simulink model "Control"  (R2022b)
settings: Solver=ode4  StartTime=0.0  StopTime=60  FixedStep=0.001  RelTol=1e-3
undefined symbols (not defined in the file): Am, gv, iPhi, NC, NCP, nodeControl, nodeDisturbe, Psi1, Psi2, V0, W1, W2
settings Model: Creator=raul  LastModifiedBy=raul

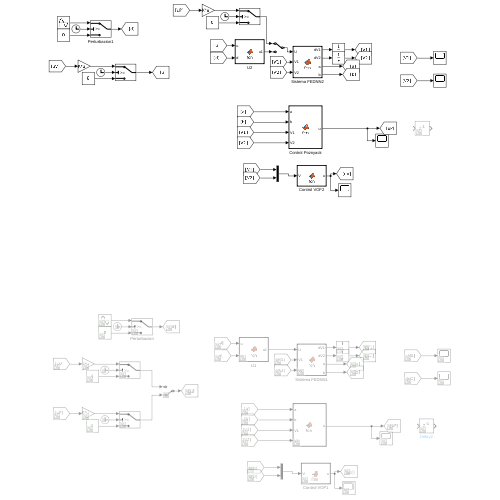
[thumbnail: Simulink's stored preview of the top-level diagram]
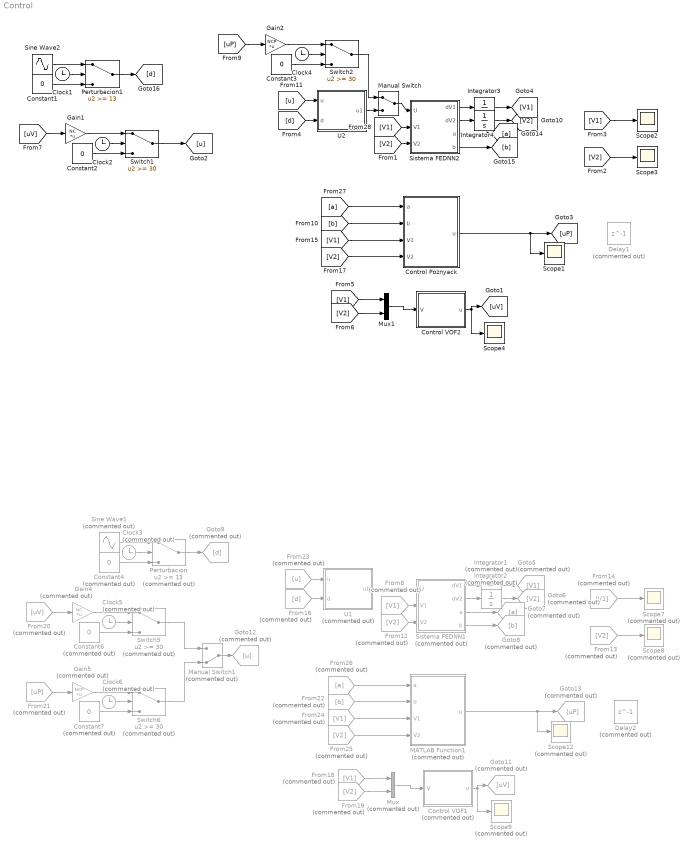
== system Control ==
  Clock1 : Clock
  Clock2 : Clock
  Clock3 : Clock  Commented=on
  Clock4 : Clock
  Clock5 : Clock  Commented=on
  Clock6 : Clock  Commented=on
  Constant1 : Constant  Value=0
  Constant2 : Constant  Value=0
  Constant3 : Constant  Value=0
  Constant4 : Constant  Commented=on  Value=0
  Constant6 : Constant  Commented=on  Value=0
  Constant7 : Constant  Commented=on  Value=0
  Control Poznyack : MATLAB Function  TreatAsAtomicUnit=on
  Control VOF1 : MATLAB Function  Commented=on  TreatAsAtomicUnit=on
  Control VOF2 : MATLAB Function  TreatAsAtomicUnit=on
  Delay1 : Delay  Commented=on  DelayLength=1  InitialCondition=zeros(20,1)
  Delay2 : Delay  Commented=on  DelayLength=1  InitialCondition=zeros(20,1)
  From{12..13,19,25} (4 alike) : From  Commented=on  GotoTag=V2
  From{8,14,18,24} (4 alike) : From  Commented=on  GotoTag=V1
  From16 : From  Commented=on  GotoTag=d
  From20 : From  Commented=on  GotoTag=uV
  From21 : From  Commented=on  GotoTag=uP
  From22 : From  Commented=on  GotoTag=b
  From23 : From  Commented=on  GotoTag=u
  From26 : From  Commented=on  GotoTag=a
  Gain1 : Gain  Gain=NC  Multiplication=Matrix(K*u)
  Gain2 : Gain  Gain=NCP  Multiplication=Matrix(K*u)
  Gain4 : Gain  Commented=on  Gain=NC  Multiplication=Matrix(K*u)
  Gain5 : Gain  Commented=on  Gain=NCP  Multiplication=Matrix(K*u)
  Goto11 : Goto  Commented=on  GotoTag=uV
  Goto12 : Goto  Commented=on  GotoTag=u
  Goto13 : Goto  Commented=on  GotoTag=uP
  Goto5 : Goto  Commented=on  GotoTag=V1
  Goto6 : Goto  Commented=on  GotoTag=V2
  Goto7 : Goto  Commented=on  GotoTag=a
  Goto8 : Goto  Commented=on  GotoTag=b
  Goto9 : Goto  Commented=on  GotoTag=d
  Integrator1 : Integrator  Commented=on  InitialCondition=V0(1:20)
  Integrator2 : Integrator  Commented=on  InitialCondition=V0(21:40)
  Integrator3 : Integrator  InitialCondition=V0(1:20)
  Integrator4 : Integrator  InitialCondition=V0(21:40)
  MATLAB Function1 : MATLAB Function  Commented=on  TreatAsAtomicUnit=on
  Manual Switch : ManualSwitch
  Manual Switch1 : ManualSwitch  Commented=on  CurrentSetting=0
  Mux : Mux  Commented=on  Inputs=2
  Mux1 : Mux  Inputs=2
  Perturbacion : Switch  Commented=on  Threshold=13  SaturateOnIntegerOverflow=off  InputSameDT=off
  Perturbacion1 : Switch  Threshold=13  SaturateOnIntegerOverflow=off  InputSameDT=off
  Scope{1..4} (4 alike) : Scope
  Scope{7..9,12} (4 alike) : Scope  Commented=on
  Sine Wave1 : Sin  Commented=on  SampleTime=0
  Sine Wave2 : Sin  SampleTime=0
  Sistema FEDNN1 : MATLAB Function  Commented=on  TreatAsAtomicUnit=on
  Sistema FEDNN2 : MATLAB Function  TreatAsAtomicUnit=on
  Switch1 : Switch  Threshold=30  SaturateOnIntegerOverflow=off  InputSameDT=off
  Switch2 : Switch  Threshold=30  SaturateOnIntegerOverflow=off  InputSameDT=off
  Switch5 : Switch  Commented=on  Threshold=30  SaturateOnIntegerOverflow=off  InputSameDT=off
  Switch6 : Switch  Commented=on  Threshold=30  SaturateOnIntegerOverflow=off  InputSameDT=off
  U1 : MATLAB Function  Commented=on  TreatAsAtomicUnit=on
  U2 : MATLAB Function  TreatAsAtomicUnit=on
  wires:
  Sistema FEDNN1/1(dV1) -> Integrator1/1
  Integrator1/1 -> Goto5/1
  From8/1 -> Sistema FEDNN1/2(V1)
  Integrator2/1 -> Goto6/1
  Sistema FEDNN1/2(dV2) -> Integrator2/1
  From12/1 -> Sistema FEDNN1/3(V2)
  Sistema FEDNN1/3(a) -> Goto7/1
  Sistema FEDNN1/4(b) -> Goto8/1
  From14/1 -> Scope7/1
  From13/1 -> Scope8/1
  Clock3/1 -> Perturbacion/2
  Sine Wave1/1 -> Perturbacion/1
  Constant4/1 -> Perturbacion/3
  Perturbacion/1 -> Goto9/1
  Mux/1 -> Control VOF1/1(V)
  Control VOF1/1(u) -> Goto11/1, Scope9/1
  From18/1 -> Mux/1
  From19/1 -> Mux/2
  Clock5/1 -> Switch5/2
  Constant6/1 -> Switch5/3
  Gain4/1 -> Switch5/1
  From20/1 -> Gain4/1
  From16/1 -> U1/2(d)
  From23/1 -> U1/1(u)
  From26/1 -> MATLAB Function1/1(a)
  From25/1 -> MATLAB Function1/4(V2)
  From24/1 -> MATLAB Function1/3(V1)
  From22/1 -> MATLAB Function1/2(b)
  Clock6/1 -> Switch6/2
  Constant7/1 -> Switch6/3
  Gain5/1 -> Switch6/1
  From21/1 -> Gain5/1
  U1/1(u1) -> Sistema FEDNN1/1(U)
  Manual Switch1/1 -> Goto12/1
  Switch5/1 -> Manual Switch1/1
  Switch6/1 -> Manual Switch1/2
  MATLAB Function1/1(u) -> Scope12/1, Goto13/1
  [V1] -> Control Poznyack/3(V1)
  [uP] -> Gain2/1
  Constant3/1 -> Switch2/3
  [a] -> Control Poznyack/1(a)
  [b] -> Control Poznyack/2(b)
  Gain1/1 -> Switch1/1
  Clock1/1 -> Perturbacion1/2
  [d] -> U2/2(d)
  Constant2/1 -> Switch1/3
  Sistema FEDNN2/1(dV1) -> Integrator3/1
  Clock2/1 -> Switch1/2
  [V2] -> Control Poznyack/4(V2)
  Mux1/1 -> Control VOF2/1(V)
  [V2] -> Mux1/2
  Sistema FEDNN2/3(a) -> [a]
  [V2] -> Sistema FEDNN2/3(V2)
  Sistema FEDNN2/4(b) -> [b]
  Constant1/1 -> Perturbacion1/3
  [V2] -> Scope3/1
  Control Poznyack/1(u) -> Scope1/1, [uP]
  Sine Wave2/1 -> Perturbacion1/1
  Perturbacion1/1 -> [d]
  [u] -> U2/1(u)
  [V1] -> Mux1/1
  [V1] -> Sistema FEDNN2/2(V1)
  Integrator4/1 -> [V2]
  Control VOF2/1(u) -> [uV], Scope4/1
  Integrator3/1 -> [V1]
  [uV] -> Gain1/1
  Sistema FEDNN2/2(dV2) -> Integrator4/1
  [V1] -> Scope2/1
  Gain2/1 -> Switch2/1
  Clock4/1 -> Switch2/2
  Switch1/1 -> [u]
  U2/1(u1) -> Manual Switch/2
  Manual Switch/1 -> Sistema FEDNN2/1(U)
  Switch2/1 -> Manual Switch/1

== matlab function Control/MATLAB Function1 ==
  data: a input; u output; b input; k parameter; V1 input; V2 input
function u = fcn(a, b, k, V1, V2)
    epsilon = 1; % Regularización pequeña
    b_reg = b + epsilon * eye(size(b)); % Regularización con epsilon pequeño

    z = V1;
    y = V2;

    miu = -k * y;

    % Usar pseudo-inversa para mayor estabilidad
%     binv=pinv(b_reg);
    u = (miu-z-a) ;
    
    
%     tol = 1e-10;


%     % Verifica si el determinante es mayor que la tolerancia
%     if abs(det()) > tol
%         inver = 1; % La matriz es invertible
%     else
%         inver = 0; % La matriz no es invertible
%     end

end

== matlab function Control/Control VOF2 ==
  data: V input; u output; gv parameter; iPhi parameter
function u = fcn(V,gv,iPhi)


y=iPhi*V;

u=-gv*y;

== matlab function Control/Control Poznyack ==
  data: a input; u output; b input; k parameter; V1 input; V2 input
function u = fcn(a, b, k, V1, V2)
    epsilon = 1; % Regularización pequeña
    b_reg = b + epsilon * eye(size(b)); % Regularización con epsilon pequeño

    z = V1;
    y = V2;

    miu = -k * y;

    % Usar pseudo-inversa para mayor estabilidad
%     binv=pinv(b_reg);
    u = pinv(b_reg)*(miu-z-a) ;
    
    
%     tol = 1e-10;


%     % Verifica si el determinante es mayor que la tolerancia
%     if abs(det()) > tol
%         inver = 1; % La matriz es invertible
%     else
%         inver = 0; % La matriz no es invertible
%     end

end

== matlab function Control/Sistema FEDNN1 ==
  data: U input; V1 input; V2 input; W1 parameter; W2 parameter; Psi1 parameter; Psi2 parameter; Am parameter; dV1 output; dV2 output; a output; b output
function [dV1,dV2,a,b] = fcn(U,V1,V2, W1, W2, Psi1, Psi2, Am)

V=[V1;V2];
a=Am*V+W1*sigmoid(Psi1,V);
b=W2*phi_sigmoid(Psi2,V);

dV1=V2;
dV2=a+b*U;



function s = sigmoid(b,x)
   s = 1./(1+exp(-b*x)); 
end



function phi = phi_sigmoid(bp, xp)
    % Comprueba que b y x tengan las dimensiones adecuadas
    [rows_b, cols_b] = size(bp);
    [rows_x, cols_x] = size(xp);

    % Inicializa la matriz de salida
    phi = zeros(rows_b, rows_b); % Matriz de 20x20

    % Calcula la sigmoide combinando cada fila de b con el vector x
    for i = 1:rows_b
        phi(i, :) = 1 ./ (1 + exp(-bp(i, :) * xp)); % Producto y sigmoide
    end
end



end

== matlab function Control/Sistema FEDNN2 ==
  data: U input; V1 input; V2 input; W1 parameter; W2 parameter; Psi1 parameter; Psi2 parameter; Am parameter; dV1 output; dV2 output; a output; b output
function [dV1,dV2,a,b] = fcn(U,V1,V2, W1, W2, Psi1, Psi2, Am)

V=[V1;V2];
a=Am*V+W1*sigmoid(Psi1,V);
b=W2*phi_sigmoid(Psi2,V);

dV1=V2;
dV2=a+b*U;



function s = sigmoid(b,x)
   s = 1./(1+exp(-b*x)); 
end



function phi = phi_sigmoid(bp, xp)
    % Comprueba que b y x tengan las dimensiones adecuadas
    [rows_b, cols_b] = size(bp);
%     [rows_x, cols_x] = size(xp);

    % Inicializa la matriz de salida
    phi = zeros(rows_b, rows_b); % Matriz de 20x20

    % Calcula la sigmoide combinando cada fila de b con el vector x
    for i = 1:rows_b
        phi(i, :) = 1 ./ (1 + exp(-bp(i, :) * xp)); % Producto y sigmoide
    end
end



end

== matlab function Control/U1 ==
  data: u1 output; u input; d input; nodeControl parameter; nodeDisturbe parameter
function u1 = fcn(u, d, nodeControl, nodeDisturbe)%add Bw,w

u1=zeros(20,1);
u1(nodeDisturbe,1)=d;
u1(nodeControl,1)=u;

== matlab function Control/U2 ==
  data: u1 output; u input; d input; nodeControl parameter; nodeDisturbe parameter
function u1 = fcn(u, d, nodeControl, nodeDisturbe)%add Bw,w

u1=zeros(20,1);
u1(nodeDisturbe,1)=d;
u1(nodeControl,1)=u;

== matlab function Control/Control VOF1 ==
  data: V input; u output; gv parameter; iPhi parameter
function u = fcn(V,gv,iPhi)


y=iPhi*V;

u=-gv*y;
